simulink model "week2_4"  (R2020b)
settings: Solver=VariableStepAuto  StartTime=0.0  StopTime=10.0  RelTol=1e-3
model workspace (MAT data in the model file):
  J = Simulink.Parameter
  J.Value = 3.2284e-06
  J.DataType = 'auto'
  J.Dimensions = [1 1]
  K = Simulink.Parameter
  K.Value = 0.0274
  K.DataType = 'auto'
  K.Dimensions = [1 1]
  Ke = Simulink.Parameter
  Ke.Value = 0.0274
  Ke.DataType = 'auto'
  Ke.Dimensions = [1 1]
  Kt = Simulink.Parameter
  Kt.Value = 0.0274
  Kt.DataType = 'auto'
  Kt.Dimensions = [1 1]
  L = Simulink.Parameter
  L.Value = 2.75e-06
  L.DataType = 'auto'
  L.Dimensions = [1 1]
  R = Simulink.Parameter
  R.Value = 4
  R.DataType = 'auto'
  R.Dimensions = [1 1]
  b = Simulink.Parameter
  b.Value = 3.5077e-06
  b.DataType = 'auto'
  b.Dimensions = [1 1]
settings Model: Creator=lalit  LastModifiedBy=lalit

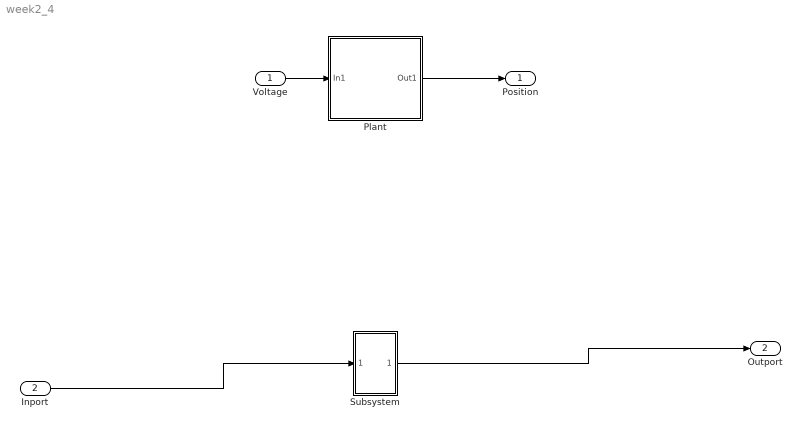
== system week2_4 ==
  Voltage : Inport
  Inport : Inport  Port=2
  Plant : Subsystem
  Subsystem : ModelReference  ModelNameDialog=PIcontoller  SimulationMode=Normal  ModelReferenceVersion=1.18
  Position : Outport
  Outport : Outport  Port=2
  wires:
  Voltage/1 -> Plant/1(In1)
  Plant/1(Out1) -> Position/1
  Inport/1 -> Subsystem/1
  Subsystem/1 -> Outport/1

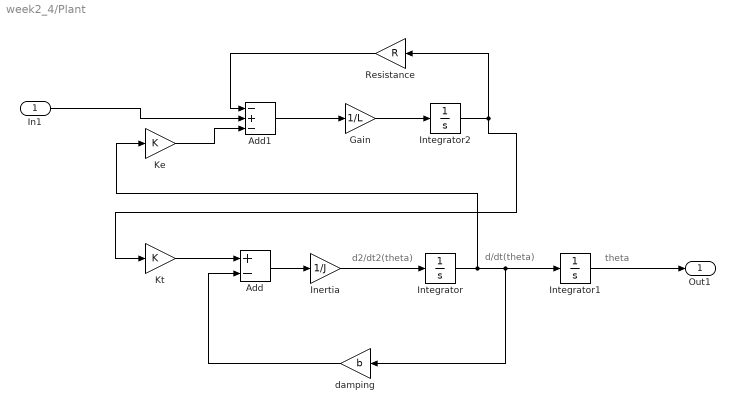
== system week2_4/Plant ==
  note: theta
  note: d2/dt2(theta)
  note: d/dt(theta)
  In1 : Inport
  Add : Sum  Inputs=+-
  Add1 : Sum  Inputs=-+-
  Gain : Gain  Gain=1/L
  Inertia : Gain  Gain=1/J
  Integrator : Integrator
  Integrator1 : Integrator
  Integrator2 : Integrator
  Ke : Gain  Gain=K
  Kt : Gain  Gain=K
  Resistance : Gain  Gain=R
  damping : Gain  Gain=b
  Out1 : Outport
  wires:
  Resistance/1 -> Add1/1
  Add1/1 -> Gain/1
  Kt/1 -> Add/1
  Integrator/1 -> Ke/1, damping/1, Integrator1/1
  Ke/1 -> Add1/3
  Integrator2/1 -> Kt/1, Resistance/1
  Gain/1 -> Integrator2/1
  Add/1 -> Inertia/1
  damping/1 -> Add/2
  Inertia/1 -> Integrator/1
  In1/1 -> Add1/2
  Integrator1/1 -> Out1/1
